simulink model "Opgave11_1"  (R2024a)
settings: Solver=VariableStepAuto  StartTime=0.0  StopTime=300  RelTol=1e-3
values from neighbouring files (symbols this model uses):
  A = [0 1; 0 -alpha]    [Kladefil.m]    (also in Opgaver.m = [-15 -6.75 -2.5)
  B = [0;1]    [Kladefil.m]    (also in Opgaver.m = [8)
  C = [K2 0]    [Kladefil.m]    (also in Opgaver.m = [0 1.5625 3.9063])
  K = [-0.9 -0.5813 -0.2031]    [Opgaver.m]
  Ke = 0.01    [Opgaver.m]
  L = [4.88 ... (first row only)    [Opgaver.m]
settings Model: Creator=jesperbertelsen  LastModifiedBy=jesperbertelsen

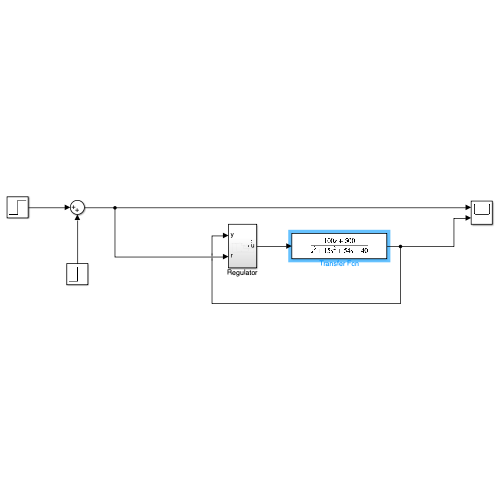
[thumbnail: Simulink's stored preview of the top-level diagram]
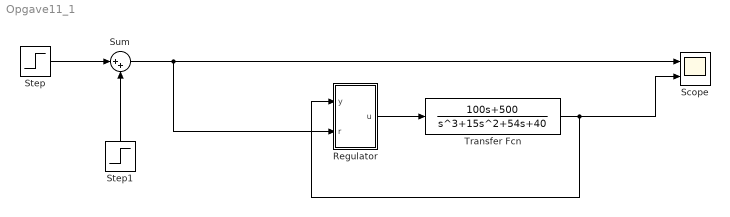
== system Opgave11_1 ==
  Regulator : Subsystem
  Scope : Scope  NumInputPorts=2
  Step : Step  After=4  SampleTime=0
  Step1 : Step  Time=40  After=4  SampleTime=0
  Sum : Sum  Inputs=|++
  Transfer Fcn : TransferFcn  Numerator=[100 500]  Denominator=[1 15 54 40]
  wires:
  Step/1 -> Sum/1
  Step1/1 -> Sum/2
  Sum/1 -> Regulator/2(r), Scope/1
  Transfer Fcn/1 -> Regulator/1(y), Scope/2
  Regulator/1(u) -> Transfer Fcn/1

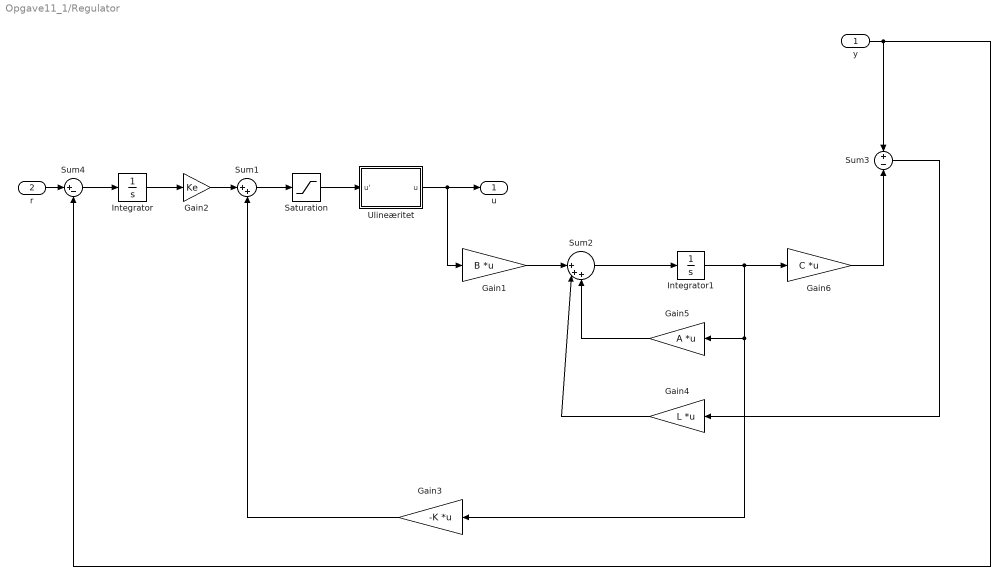
== system Opgave11_1/Regulator ==
  y : Inport
  r : Inport  Port=2
  Gain1 : Gain  Gain=B  Multiplication=Matrix(K*u)
  Gain2 : Gain  Gain=Ke
  Gain3 : Gain  Gain=-K  Multiplication=Matrix(K*u)
  Gain4 : Gain  Gain=L  Multiplication=Matrix(K*u)
  Gain5 : Gain  Gain=A  Multiplication=Matrix(K*u)
  Gain6 : Gain  Gain=C  Multiplication=Matrix(K*u)
  Integrator : Integrator
  Integrator1 : Integrator
  Saturation : Saturate  UpperLimit=1  LowerLimit=-1
  Sum1 : Sum  Inputs=|++
  Sum2 : Sum  Inputs=||+++
  Sum3 : Sum  Inputs=+|-
  Sum4 : Sum  Inputs=|+-
  Ulineæritet : Subsystem
  u : Outport
  wires:
  r/1 -> Sum4/1
  Gain5/1 -> Sum2/3
  Sum2/1 -> Integrator1/1
  Gain4/1 -> Sum2/2
  Gain6/1 -> Sum3/2
  Integrator1/1 -> Gain3/1, Gain5/1, Gain6/1
  Gain3/1 -> Sum1/2
  Sum4/1 -> Integrator/1
  y/1 -> Sum3/1, Sum4/2
  Sum3/1 -> Gain4/1
  Gain1/1 -> Sum2/1
  Sum1/1 -> Saturation/1
  Ulineæritet/1(u) -> u/1, Gain1/1
  Saturation/1 -> Ulineæritet/1(u')
  Integrator/1 -> Gain2/1
  Gain2/1 -> Sum1/1

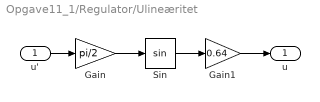
== system Opgave11_1/Regulator/Ulineæritet ==
  u' : Inport
  Gain : Gain  Gain=pi/2
  Gain1 : Gain  Gain=0.64
  Sin : Trigonometry
  u : Outport
  wires:
  u'/1 -> Gain/1
  Sin/1 -> Gain1/1
  Gain/1 -> Sin/1
  Gain1/1 -> u/1
